simulink model "heli_close"  (R2021a)
settings: Solver=VariableStepAuto  StartTime=0.0  StopTime=10  FixedStep=0.001  RelTol=1e-3
values from neighbouring files (symbols this model uses):
  A = [-0.4 0 -0.01 ... (first row only)    [heli.m]
  B = [6.3 0 9.8]'    [heli.m]
  C = [0 0 1]    [heli.m]
  K = [eval(KSO.K1) eval(KSO.K2) eval(KSO.K3)]    [heli.m]
settings Model: Creator=McQueen_Zero  LastModifiedBy=McQueen_Zero
settings OptimizationCC: DefaultParameterBehavior=Inlined  BufferReuse=off
settings DebuggingCC: InitInArrayFormatMsg=none

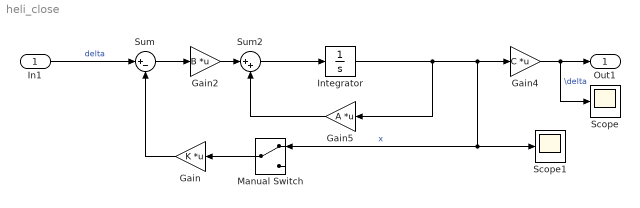
== system heli_close ==
  In1 : Inport
  Gain : Gain  Gain=K  Multiplication=Matrix(K*u)
  Gain2 : Gain  Gain=B  Multiplication=Matrix(K*u)
  Gain4 : Gain  Gain=C  Multiplication=Matrix(K*u)
  Gain5 : Gain  Gain=A  Multiplication=Matrix(K*u)
  Integrator : Integrator
  Manual Switch : ManualSwitch
  Scope : Scope
  Scope1 : Scope
  Sum : Sum  Inputs=|+-
  Sum2 : Sum  Inputs=|++
  Out1 : Outport
  wires:
  Integrator/1 -> Gain4/1, Manual Switch/1, Scope1/1, Gain5/1  "x"
  In1/1 -> Sum/1  "delta"
  Manual Switch/1 -> Gain/1
  Gain/1 -> Sum/2
  Sum/1 -> Gain2/1
  Gain2/1 -> Sum2/1
  Sum2/1 -> Integrator/1
  Gain4/1 -> Out1/1, Scope/1  "\\delta"
  Gain5/1 -> Sum2/2
